simulink model "ex03_alarm"  (R2020b)
settings: Solver=VariableStepAuto  StartTime=0.0  StopTime=40  RelTol=1e-3
model workspace (MAT data in the model file):
  courseObject.course = 'stateflow'
  courseObject.chapter = 3
  courseObject.lesson = 3
  courseObject.section = 1
  courseObject.task = 1
undefined symbols (not defined in the file): sigbuilder_block
settings Model: PacingRate=3  Creator=gb  LastModifiedBy=19255551
settings DataIOCC: SaveTime=off

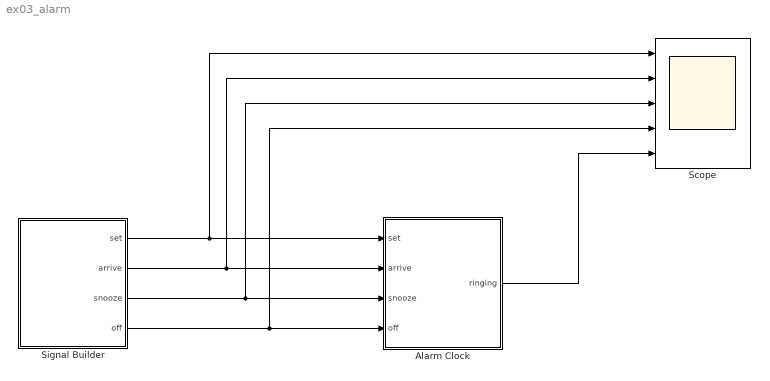
== system ex03_alarm ==
  Alarm Clock : Stateflow chart  TreatAsAtomicUnit=on
  Scope : Scope  NumInputPorts=5
  Signal Builder : Subsystem  Tag=STV Subsys  LoadFcn=sigbuilder_block('load',[6 6 1012.5 506.25 ]);  StartFcn=sigbuilder_block('start');  StopFcn=sigbuilder_block('stop');  ClipboardFcn=sigbuilder_block('clipboard');  mask(Sigbuilder block){tuvar=[0:10]}
      mask help: Simulink:masks:SigbuilderBlock_MD
      mask init:
      | if ~strcmp(get_param(bdroot(gcbh),'SimulationStatus'),'stopped') tuvar = sigbuilder_block('maskInit'); end
      settings: CopyFcn=sigbuilder_block('copy');  DeleteFcn=sigbuilder_block('delete');  ModelCloseFcn=sigbuilder_block('modelClose');  PreSaveFcn=sigbuilder_block('preSave');  PauseFcn=sigbuilder_block('pause');  ContinueFcn=sigbuilder_block('continue');  NameChangeFcn=sigbuilder_block('namechange');  OpenFcn=sigbuilder_block('open',[4.8 4.8 1142.4 586.8 ]);  CloseFcn=sigbuilder_block('close');
      mask Display: plot(0, 0, 100, 100,[2, 2, 32, 32, 2], [68, 8, 8, 68, 68],[32, 2], [38, 38], [32, 19, 2],[53, 60, 44], [32, 17, 17, 2],[16, 16, 31, 31]);txt = getActiveGroup(gcbh);text(2, 100, txt,'verticalAlignment', 'top');
  wires:
  Signal Builder/3(snooze) -> Scope/3, Alarm Clock/3(snooze)
  Signal Builder/2(arrive) -> Scope/2, Alarm Clock/2(arrive)
  Signal Builder/1(set) -> Scope/1, Alarm Clock/1(set)
  Alarm Clock/1(ringing) -> Scope/5
  Signal Builder/4(off) -> Alarm Clock/4(off), Scope/4

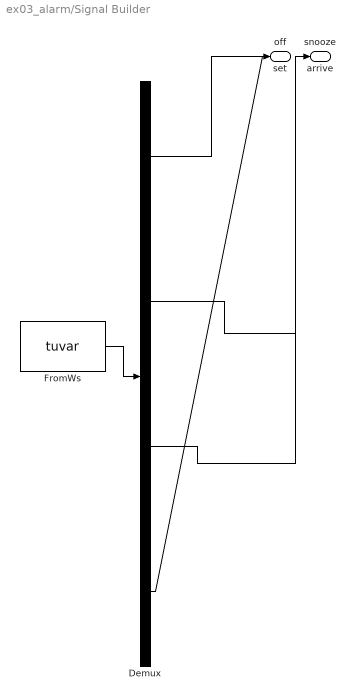
== system ex03_alarm/Signal Builder ==
  Demux : Demux  Tag=STV Demux
      settings: DisplayOption=none
  FromWs : FromWorkspace  Tag=STV FromWs  VariableName=tuvar
      SigBuilderData=|
      | common.afterFinalStr = 'Extrapolate'
      | common.sampleTime = 0
      | dataSet.timeRange = [0 20]
      | dataSet.name = 'Group 1'
      | sbobj.Groups.Name = 'Group 1'
      | sbobj.Groups.Signals(1).Name = 'set'
      | sbobj.Groups.Signals(1).XData = [0 0.5 0.5 1 1 10 10 10.5 10.5 20]
      | sbobj.Groups.Signals(1).YData = [0 0 1 1 0 0 1 1 0 0]
      | sbobj.Groups.Signals(2).Name = 'arrive'
      | sbobj.Groups.Signals(2).XData = [0 2 2 2.5 2.5 4.5 4.5 5 5 11 11 11.5 11.5 20]
      | sbobj.Groups.Signals(2).YData = [0 0 1 1 0 0 1 1 0 0 1 1 0 0]
      | sbobj.Groups.Signals(3).Name = 'snooze'
      | sbobj.Groups.Signals(3).XData = [0 3 3 3.5 3.5 5.5 5.5 6 6 20]
      | sbobj.Groups.Signals(3).YData = [0 0 1 1 0 0 1 1 0 0]
      | sbobj.Groups.Signals(4).Name = 'off'
      | sbobj.Groups.Signals(4).XData = [0 7.5 7.5 8 8 20]
      | sbobj.Groups.Signals(4).YData = [0 0 1 1 0 0]
      | sbobj.Groups.TimeRange = [0 20]
  set : Outport  Tag=STV Outport
  arrive : Outport  Tag=STV Outport  Port=2
  snooze : Outport  Tag=STV Outport  Port=3
  off : Outport  Tag=STV Outport  Port=4
  wires:
  FromWs/1 -> Demux/1
  Demux/1 -> set/1
  Demux/2 -> arrive/1
  Demux/3 -> snooze/1
  Demux/4 -> off/1

== stateflow chart ex03_alarm/Alarm Clock ==
  state alarm
    state ringing
      entry:
      ringing = 1;
    state start
      entry:
      ringing = 0;
    state snooze
      entry:
      ringing = 0;
    state set
      entry:
    (default) -> start
    ringing -> start [order 3] : [off == 0]
    ringing -> start [order 2] : after(10,sec)
    snooze -> start [order 2] : [off == 0]
    set -> ringing [order 1] : [arrive == 1]
    set -> start [order 2] : [off == 0]
    start -> set : [set == 1]
    ringing -> snooze [order 1] : [snooze == 1]
    snooze -> ringing [order 1] : [arrive == 1]
  (default) -> alarm
  data: set input; arrive input; snooze input; off input; ringing output
